simulink model "ex2model2022a"  (R2022b)
settings: Solver=FixedStepAuto  StartTime=0.0  StopTime=30  FixedStep=0.0001  RelTol=1e-3
values from neighbouring files (symbols this model uses):
  a21 = 1/(2*m)*x30^2*FemP1/FemP2^2*exp(-x10/FemP2)    [ex4.m]
  a23 = -1/(m)*x30*FemP1/FemP2*exp(-x10/FemP2)    [ex4.m]
  a31 = 1/f1*exp(x10/f2)*(ki*u10+ci-x30)    [ex4.m]
  a33 = -f2/f1*exp(x10/f2)    [ex4.m]
  b31 = ki*f2/f1*exp(x10/f2)    [ex4.m]
  g = 9.81    [ex4.m]
  k = -place(A, B(:,1), -s)    [ex4.m]
settings Model: Creator=AgraWoodAdmin  LastModifiedBy=MPatr
settings DebuggingCC: UnconnectedInputMsg=warning  UnconnectedOutputMsg=warning  UnconnectedLineMsg=warning
settings ModelReferenceCC: EnableRefExpFcnMdlSchedulingChecks=on
settings RTWCC: DLArmComputeVersion=19.05

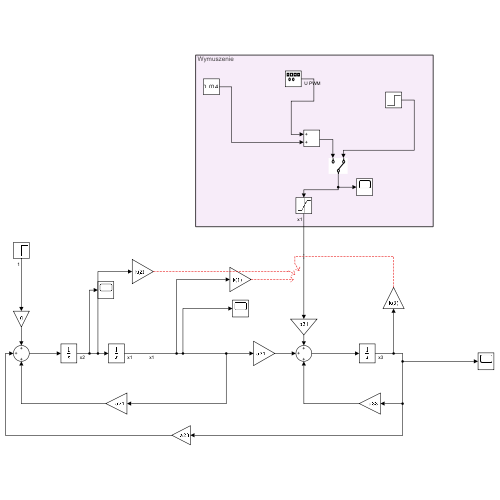
[thumbnail: Simulink's stored preview of the top-level diagram]
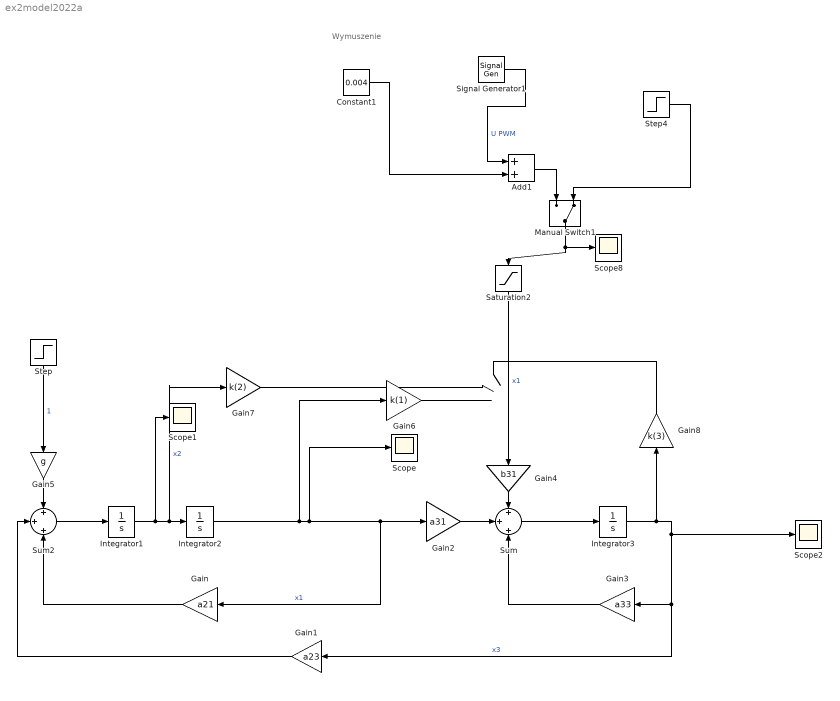
== system ex2model2022a ==
  note: Wymuszenie
  Add1 : Sum
  Constant1 : Constant  Value=0.004
  Gain : Gain  Gain=a21
  Gain1 : Gain  Gain=a23
  Gain2 : Gain  Gain=a31
  Gain3 : Gain  Gain=a33
  Gain4 : Gain  Gain=b31
  Gain5 : Gain  Gain=g
  Gain6 : Gain  Gain=k(1)
  Gain7 : Gain  Gain=k(2)
  Gain8 : Gain  Gain=k(3)
  Integrator1 : Integrator
  Integrator2 : Integrator
  Integrator3 : Integrator
  Manual Switch1 : ManualSwitch  CurrentSetting=0
  Saturation2 : Saturate  UpperLimit=1  LowerLimit=0
  Scope{,1..2,8} (4 alike) : Scope
  Signal Generator1 : SignalGenerator  Amplitude=.002  Units=rad/sec
  Step : Step  Time=0  SampleTime=0
  Step4 : Step  Time=0  SampleTime=0
  Sum : Sum  Inputs=+|+|+
  Sum2 : Sum  Inputs=+|+|+
  wires:
  Sum2/1 -> Integrator1/1
  Sum/1 -> Integrator3/1
  Integrator1/1 -> Scope1/1, Gain7/1, Integrator2/1  "x2"
  Integrator3/1 -> Gain8/1, Scope2/1, Gain3/1, Gain1/1  "x3"
  Gain/1 -> Sum2/3
  Gain1/1 -> Sum2/2
  Gain2/1 -> Sum/2
  Gain3/1 -> Sum/3
  Gain4/1 -> Sum/1
  Gain5/1 -> Sum2/1
  Step/1 -> Gain5/1  "1"
  Integrator2/1 -> Gain6/1, Scope/1, Gain2/1, Gain/1  "x1"
  Constant1/1 -> Add1/2
  Step4/1 -> Manual Switch1/2
  Signal Generator1/1 -> Add1/1  "U PWM"
  Add1/1 -> Manual Switch1/1
  Manual Switch1/1 -> Scope8/1, Saturation2/1
  Saturation2/1 -> Gain4/1  "x1"
  Gain6/1 -> ?
  Gain7/1 -> ?
  Gain8/1 -> ?
